simulink subsystem "PvtSubSys_VSM_ELK"  (R2020b)
settings: Solver=VariableStepAuto  StartTime=0.0  StopTime=10.0  RelTol=1e-3
values from neighbouring files (symbols this model uses):
  P_VSM_ELK_Curvature_R_Table : value not decoded    [ELK.sldd]
  P_VSM_ELK_Curvature_R_Table_Calibration : value not decoded    [ELK.sldd]
  P_VSM_ELK_Lane_Width_Table : value not decoded    [ELK.sldd]
  P_VSM_ELK_Lane_Width_Table_Calibration : value not decoded    [ELK.sldd]
  P_VSM_ELK_Lateral_Speed_Table : value not decoded    [ELK.sldd]
  P_VSM_ELK_Lateral_Speed_Table_Calibration : value not decoded    [ELK.sldd]
  P_VSM_ELK_OnComing_Lateral = 2.8    [ELK.sldd]
  P_VSM_ELK_OnComing_TTC = 3.0    [ELK.sldd]
  P_VSM_ELK_OverTaking_Lateral = 2.0    [ELK.sldd]
  P_VSM_ELK_OverTaking_TTC = 5.0    [ELK.sldd]
  P_VSM_ELK_Sensitive_Table : value not decoded    [ELK.sldd]
  P_VSM_ELK_Sensitive_Table_Calibration : value not decoded    [ELK.sldd]
  P_VSM_ELK_State_Absesp_enable = 1.0    [ELK.sldd]
  P_VSM_ELK_State_Accpedalrate_enable = 1.0    [ELK.sldd]
  P_VSM_ELK_State_Breakpressure_enable = 1.0    [ELK.sldd]
  P_VSM_ELK_State_DriverInputTrqValue_enable = 1.0    [ELK.sldd]
  P_VSM_ELK_State_Eps_enable = 1.0    [ELK.sldd]
  P_VSM_ELK_State_ESSSts_enable = 1.0    [ELK.sldd]
  P_VSM_ELK_State_Failsafe_enable = 1.0    [ELK.sldd]
  P_VSM_ELK_State_GEAR_enable = 1.0    [ELK.sldd]
  P_VSM_ELK_State_Handson_enable = 1.0    [ELK.sldd]
  P_VSM_ELK_State_Headingangle_enable = 1.0    [ELK.sldd]
  P_VSM_ELK_State_Lane_enable = 1.0    [ELK.sldd]
  P_VSM_ELK_State_LaneChange_enable = 1.0    [ELK.sldd]
  P_VSM_ELK_State_Lanecurve_enable = 1.0    [ELK.sldd]
  P_VSM_ELK_State_LateralAcce_enable = 1.0    [ELK.sldd]
  P_VSM_ELK_State_LongitudeAcc_enable = 1.0    [ELK.sldd]
  P_VSM_ELK_State_Overide_enable = 1.0    [ELK.sldd]
  P_VSM_ELK_State_Param_AngleOffset = 0.05    [ELK.sldd]
  P_VSM_ELK_State_Param_LaneTime : value not decoded    [ELK.sldd]
  P_VSM_ELK_State_Param_Oncoming = 0.55    [ELK.sldd]
  P_VSM_ELK_State_Param_OnTime : value not decoded    [ELK.sldd]
  P_VSM_ELK_State_Param_OutOffset = 0.15    [ELK.sldd]
  P_VSM_ELK_State_Param_Over = 0.55    [ELK.sldd]
  P_VSM_ELK_State_Param_OvTime : value not decoded    [ELK.sldd]
  P_VSM_ELK_State_Param_Speed : value not decoded    [ELK.sldd]
  P_VSM_ELK_State_SteerWheelAngle_enable = 1.0    [ELK.sldd]
  P_VSM_ELK_State_SteerWheelSpd_enable = 1.0    [ELK.sldd]
  P_VSM_ELK_State_TurnLight_enable = 1.0    [ELK.sldd]
  P_VSM_ELK_State_Vehspeed_enable = 1.0    [ELK.sldd]
  P_VSM_ELK_State_Yawsup_enable = 1.0    [ELK.sldd]
undefined symbols (not defined in the file or in its folder): ELKSTATE, P_Global_DxvRearBumper_m, P_Global_IEnvironment_RefPX_Front_Bumper, P_Global_IFV2Fwheel_Dx, P_Global_Vehicle_Length_m, P_Global_VehicleWidthMin_m, P_VSM_LSMC_SampleTime
libraries: simulink x167
(part 5 of 5)

== matlab function PvtSubSys_VSM_ELK/ELK_OnComing_OverTaking/OverTaking/Left_tar ==
  data: v_t output; dx input; id input; inID input; vx input; x output; minid output; la_offset input; offset output; Vehicle_Length input
function [v_t,x,minid,offset] = fcn(dx,id,inID,vx,la_offset,Vehicle_Length)%借鉴BSD
t_x=single(ones(8,1)*(-520));
t=single(0);
v_t=single(0);
x=single(-520);
minid=uint8(0);
offset=single(520);
for i=1:8          % dy原始数据 自车左后侧 为 负值；已经改为正值。
        if    inID(i)>0   % lateral range by ID
            t_x(i)=dx(i);    % related long target
        end
end
for k=1:8
    if t_x(k)<0           % find lateral target
        t=t_x(k);
        break
    end
end
for j=1:8
    if t_x(j) >= t && t_x(j) < Vehicle_Length && t_x(j)~=-520 % after limit line
        t=t_x(j);      %min(long) target
        v_t=vx(j);
        x=dx(j);
        minid=id(j);
        offset=la_offset(j);
    end
end

== matlab function PvtSubSys_VSM_ELK/ELK_OnComing_OverTaking/OverTaking/MATLAB Function1 ==
  data: target_id input; in input; condition output single; out input; ID output; IDk1 input uint8
function [condition,ID]  = fcn(target_id,in,out,IDk1)
ID=uint8(0);
condition=single(0);
    if in>0 
        ID=target_id;
        condition=single(1);
    elseif out>0
        ID=uint8(0);
        condition=single(0);
    elseif in==0 && out==0
        if target_id==IDk1 && target_id>0 
            condition=single(1);
            ID=IDk1;
        end
    end

== matlab function PvtSubSys_VSM_ELK/ELK_OnComing_OverTaking/OverTaking/MATLAB Function7 ==
  data: target_id input; in input; condition output single; out input; ID output; IDk1 input uint8
function [condition,ID]  = fcn(target_id,in,out,IDk1)
ID=uint8(0);
condition=single(0);
    if in>0 
        ID=target_id;
        condition=single(1);
    elseif out>0
        ID=uint8(0);
        condition=single(0);
    elseif in==0 && out==0
        if target_id==IDk1 && target_id>0 
            condition=single(1);
            ID=IDk1;
        end
    end

== matlab function PvtSubSys_VSM_ELK/ELK_OnComing_OverTaking/OverTaking/Min_Leftcar ==
  data: v input; v_t input; condition input; leftcar output; Vo1 output; x input; TTC output; la input; T input
function [leftcar,Vo1,TTC] = fcn(v,v_t,condition,x,la,T)%借鉴BSD

if   v_t~=single(0)  %  target car is moving  (in same direction)

    Vo1=v_t-v+v;  %vx 一直都是正数，vx为目标车
    TTC=(-x)/Vo1;  % 在自车后  dx是负值

    if (Vo1>0 && TTC<T && la ) || (condition > 0 && la) 
        leftcar=true;
    else
        leftcar=false;  
    end
else
    leftcar=false;
    Vo1=single(0);
    
    TTC=single(0);
end

== matlab function PvtSubSys_VSM_ELK/ELK_OnComing_OverTaking/OverTaking/Min_Reftcar ==
  data: v input; v_t input; condition input; rightcar output; Vo1 output; x input; TTC output; la input; T input
function [rightcar,Vo1,TTC] = fcn(v,v_t,condition,x,la,T)%借鉴BSD
if   v_t~=single(0)  %  target car is moving  (in same direction)

    Vo1=v_t-v+v;  %vx 一直都是正数，vx为目标车
    TTC=(-x)/Vo1;  % 在自车后  dx是负值

    if (Vo1>0 && TTC<T && la ) || (condition > 0 && la)  
        rightcar=true;
    else
        rightcar=false;  
    end
else
    rightcar=false;
    Vo1=single(0);
    
    TTC=single(0);
end

== stateflow chart PvtSubSys_VSM_ELK/ELK_OnComing_OverTaking/OverTaking/OVERTAKING_FUNCTION ==
  state OVERTAKING
    en:over_intervention=0;
  state LEFT_OVERTAKING
    en:over_intervention=1;
    LEFT_OVERTAKING -> (junction 21) [order 1]
    (junction 21) -> LEFT_OVERTAKING [order 1] : [Ldeactive]{left_count = left_count + 1;}
    (junction 21) -> LEFT_OVERTAKING [order 2] : {left_count=0;}
  state RIGHT_OVERTAKING
    en:over_intervention=2;
    RIGHT_OVERTAKING -> (junction 26) [order 1]
    (junction 26) -> RIGHT_OVERTAKING [order 1] : [Rdeactive]{right_count = right_count + 1;}
    (junction 26) -> RIGHT_OVERTAKING [order 2] : {right_count=0;}
  (default) -> OVERTAKING
  OVERTAKING -> LEFT_OVERTAKING [order 1] : [leftvalid>0&&BSDLCA_WL&&Lactive_para&&Triger]
  LEFT_OVERTAKING -> OVERTAKING [order 1] : [leftvalid==0||left_count>50||ELKState<3]{left_count=0;}
  OVERTAKING -> RIGHT_OVERTAKING [order 2] : [rightvalid>0&&BSDLCA_WR&&Ractive_para&&Triger]
  RIGHT_OVERTAKING -> OVERTAKING [order 1] : [rightvalid==0||right_count>50||ELKState<3]{right_count=0;}
  data: BSDLCA_WL input; BSDLCA_WR input; leftvalid input; rightvalid input; over_intervention output; Lactive_para input; Ractive_para input; Ldeactive input; Rdeactive input; left_count local =0; right_count local =0; Triger input; ELKState input

== matlab function PvtSubSys_VSM_ELK/ELK_OnComing_OverTaking/OverTaking/OverTaking_Judge ==
  data: l_valid input; r_valid input; L_A0 input; L_A1 input; L_A2 input; L_A3 input; R_A0 input; left_condition output; R_A1 input; R_A2 input; R_A3 input; V input; Limit input; Rlimit input; right_condition output; T input; Ldeactive input; Rdeactive input; Out_Offset input; Angle_Offset input; LOut output; ROut output; vehicle_dy input; ifv2bum input; HalfWidth input
function [left_condition,right_condition,LOut,ROut] = fcn(l_valid,r_valid,L_A0,L_A1,L_A2,L_A3,R_A0,R_A1,R_A2,R_A3,V,...
    Limit,Rlimit,T,Ldeactive,Rdeactive,Out_Offset,Angle_Offset,vehicle_dy,ifv2bum,HalfWidth)
X=V*T;
if l_valid>0
    
   a=atan(L_A1+2*X*L_A2+3*L_A3*X^2);
%    ly=abs(cos(a)*(HalfWidth+IFV2Fwheel*tan(a)));
    if a>0
        ly=(HalfWidth+ifv2bum*tan(a))*cos(a);
    else
        ly=HalfWidth;
    end

   LY=L_A0+L_A1*X+L_A2*X^2+L_A3*X^3;
   left_condition=LY-ly-Limit-vehicle_dy;
   
   if Ldeactive>-Out_Offset && Ldeactive<Out_Offset && abs(atan(L_A1))< Angle_Offset
       LOut=true;  % steady
   else
       LOut=false;
   end       
       
else
    left_condition=single(0);
  LOut=true;
end


if r_valid>0
    
   b=atan(R_A1+2*R_A2*X+3*R_A3*X^2);
%    ry=abs(cos(b)*(HalfWidth-IFV2Fwheel*tan(b)));
    if b<0
        ry=(HalfWidth-ifv2bum*tan(b))*cos(b);
    else
        ry=HalfWidth;
    end
   RY=R_A0+R_A1*X+R_A2*X^2+R_A3*X^3;
   right_condition=RY+ry-Rlimit+vehicle_dy;
   
   if Rdeactive>-Out_Offset && Rdeactive<Out_Offset && abs(atan(R_A1))<Angle_Offset
       ROut=true;
   else
       ROut=false;
   end 
else 
    right_condition=single(0);
    ROut=true;
  
end

== matlab function PvtSubSys_VSM_ELK/ELK_OnComing_OverTaking/OverTaking/Right_tar ==
  data: v_t output; dx input; id input; inID input; vx input; x output; minid output; la_offset input; offset output; Vehicle_Length input
function [v_t,x,minid,offset] = fcn(dx,id,inID,vx,la_offset,Vehicle_Length)%借鉴BSD
t_x=single(ones(8,1)*(-520));
t=single(0);
v_t=single(0);
x=single(-520);
minid=uint8(0);
offset=single(-520);
for i=1:8            % dy原始数据 自车左后侧 为 负值；已经改为正值。
        if    inID(i)>0   % lateral range by ID
            t_x(i)=dx(i);    % related long target
        end
end
for ii=1:8
    if t_x(ii)<0           % find lateral target
        t=t_x(ii);
        break
    end
end
for j=1:8
    if t_x(j) >= t && t_x(j) < Vehicle_Length && t_x(j)~=-520
        t=t_x(j);      %min(long) target
        v_t=vx(j);
        x=dx(j);
        minid=id(j);
        offset=la_offset(j);
    end
end

== matlab function PvtSubSys_VSM_ELK/ELK_OnComing_OverTaking/OverTaking/Select_tar ==
  data: Object_ELKLeftLaneObjType input; Object_ELKRightLaneObjType input; Object_DX input; Object_DY input; Object_VX input; Object_Width input; Ego_Width input; v input; leftcar output; rightcar output; la_limit input
function [leftcar,rightcar] = fcn(Object_ELKLeftLaneObjType,Object_ELKRightLaneObjType,Object_DX,Object_DY,Object_VX,...
    Object_Width,Ego_Width,v,la_limit)%借鉴BSD


leftcar=0;
rightcar=0;

for  i=1:10
    if Object_ELKLeftLaneObjType(i)==1  %  0x1:ELKLROvertakeDisMinObj 
            vx=Object_VX(i);
            dx=Object_DX(i);
            dy=Object_DY(i)-Object_Width(i); 
            Lv_re= vx-v;
            Lttc= abs(dx/ Lv_re);
            Llateral=dy-Ego_Width;
           if  (Lttc<5 && Llateral<la_limit) || (dx>-5 && Llateral<la_limit)
               leftcar=1;
           end
        
    end
end
for j=1:10
    if Object_ELKRightLaneObjType(j)==1
            rvx=Object_VX(j);
            rdx=Object_DX(j);
            rdy=Object_DY(j)+Object_Width(j);
            
            Rv_re=rvx-v;
            Rttc=abs(rdx/Rv_re);
            Rlateral=rdy+Ego_Width;
            if (Rttc<5 && Rlateral>-la_limit) || (rdx>-5 && Rlateral>-la_limit)  %dy原始数据 在自车 右侧为正；已经统一车辆坐标系
                rightcar=1;
            end
        
    end
end

== matlab function PvtSubSys_VSM_ELK/ELK_OnComing_OverTaking/OverTaking/Select_tar2 ==
  data: Object_ELKLeftLaneObjType input; Object_ELKRightLaneObjType input; Object_DX input; Object_DY input; Object_VX input; v input; leftcar output; rightcar output; la_limit input
function [leftcar,rightcar] = fcn(Object_ELKLeftLaneObjType,Object_ELKRightLaneObjType,Object_DX,Object_DY,Object_VX,v,la_limit)%借鉴BSD
LOverTaking=0;
ROverTaking=0;
ltar=zeros(10,1);
rtar=zeros(10,1);
leftcar=0;
rightcar=0;

for  i=1:10
    if Object_ELKLeftLaneObjType(i)==1  %  0x1:ELKLROvertakeDisMinObj 
        LOverTaking=1;
        ltar(i)=i;
    end
end
for j=1:10
    if Object_ELKRightLaneObjType(j)==1
        ROverTaking=1;
        rtar(j)=j;
    end
end

if LOverTaking>0
    for l=1:10
        if ltar(l)>0                         % exit
            vx=Object_VX(l);
            dx=Object_DX(l);
            dy=Object_DY(l);
            
            Lv_re= vx-v;
           Lttc= abs(dx/ Lv_re);
           Llateral=abs(dy);
           if  (Lttc<5 && Llateral<la_limit) || (dx>-5 && Llateral<la_limit)
               leftcar=1;
           end
           
        end
    end
end
if ROverTaking>0
    for r=1:10
        if rtar(r)>0
            rvx=Object_VX(r);
            rdx=Object_DX(r);
            rdy=Object_DY(r);
            
            Rv_re=rvx-v;
            Rttc=abs(rdx/Rv_re);
            Rlateral=rdy;
            if (Rttc<5 && Rlateral>-la_limit) || (rdx>-5 && Rlateral>-la_limit)  %dy原始数据 在自车 右侧为正；已经统一车辆坐标系
                rightcar=1;
            end
        end
    end
end
